simulink model "schSimuSegway_2020b"  (R2020b)
settings: Solver=VariableStepAuto  StartTime=0.0  StopTime=tfinal  RelTol=1e-3
InitFcn:
  | disp('init inports and outports numbers');
  | in_cb=1;
  | in_cm=2;
  | in_um=3;
  | out_thb=1;
  | out_thm=2;
  | out_vb=3;
  | out_vm=4;
  | out_um=5;
  | if exist('G')~=1
  | %--------------------------------------------------
  | % valeurs des parametres par defaut
  | %--------------------------------------------------
  | disp('init default parameters');
  | time_values_cb=[0,0];
  | time_values_cm=[0,0];
  | time_values_um=[0,0];
  | tfinal=10;
  | thm_init=0*pi/180;vthm_init=0*pi/180;
  | thb_init=0*pi/180;vthb_init=0*pi/180;
  | %------------------------------------------------------------------
  | % parametres des moteurs FIT0450U d'entrainement du segway en deplacement rectiligne
  | % dans ce cas les 2 moteurs sont attaques par la meme tension d'induit Um
  | %-----------------------------------------------------------------
  | 
  | Im=2*0.0061; % inertie de 2 moteurs en sortie de reducteur, ne devrait pas etre negligable !...
  | Kem= 0.277; % rapport fcem / vitesse en sortie de reducteur :V/(rd/s)=Nm/A;
  | 
  | Kim=2 *0.277;% 2. rapport couple  en sortie de reducteur/ courant :Nm/A = V/(rd/s);
  | Rm=2.8;% resistance d'induit en ohm
  | fm=2* 0.0108;% frottement visqueux en sortie de reducteur
  | u_max=5; % tension max des moteurs
  | u_dead=0.5; % bande morte due au frottement sec en volt
  | %------------------------------------------------------------------
  | % parametres mecanique du segway
  | %-----------------------------------------------------------------
  | G=9.81; % acceleration gravite terrestre en m/s2
  | % barre
  | Mb= 0.277; %Masse segway sans batterie 277g
  | Lb =  0.056000; % distance essieu centre de masse en m
  | Ib=1e-4 ; % inertie de la barre autour de son centre de masse en Kg.m^2
  | % batterie
  | Mbat=2*0.096; %masse en Kg des 2  batteries VoltCraft 5000 de 96g chacune
  | LxBat=0.022;LyBat=2*0.036;LzBat=0.075;
  | Ibat=1/12*Mbat*(LyBat^2+LzBat^2); % inertie batt/ centre de masse batt en kg.m2
  | Lbat=0.085;%0.085; % distance essieu centre de masse Batteries
  | %roues
  | Rr=0.07; % rayon des roues en m
  | Mr=2 * 0; % masse de 2 roues, negligable
  | Ir=1/2*Rr^2*Mr; % inertie des 2 roues, =1 cylindre plein de masse Mr, de rayon Rr autour de son axe de rotation
  | I1=Ir+(Mb+Mr+Mbat)*Rr^2; %avec Batterie
  | Ieb=Ib+Ibat+Mb*Lb^2+Mbat*Lbat^2;% avec Batterie
  | 
  | 
  | end
values from neighbouring files (symbols this model uses):
  Kem = 0.277    [programme_segway_etudiant.m]
settings Model: Creator=sygorra  LastModifiedBy=sygorra
settings DataIOCC: ReturnWorkspaceOutputs=off
settings DebuggingCC: ArithmeticOperatorsInVariantConditions=warning
settings SFSimCC: CustomCodeUndefinedFunction=UseInterfaceOnly

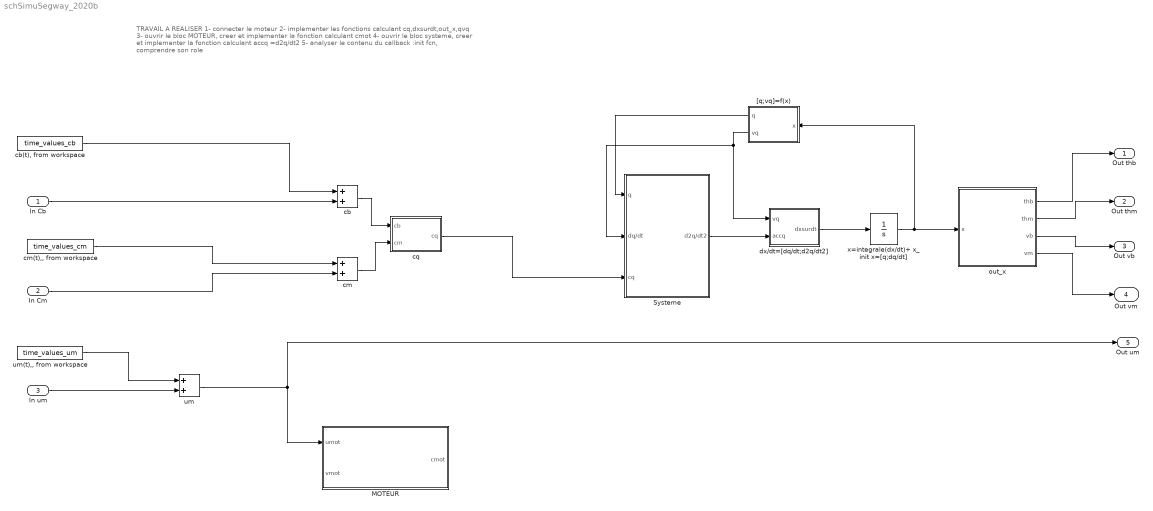
== system schSimuSegway_2020b ==
  note: TRAVAIL A REALISER
      | 1- connecter le moteur
      | 2- implementer les fonctions calculant cq,dxsurdt,out_x,qvq
      | 3- ouvrir le bloc MOTEUR, creer et implementer la fonction calculant cmot
      | 4- ouvrir le bloc systeme, creer et implementer la fonction calculant accq =d2q/dt2
      | 5- analyser le contenu du callback :init fcn, comprendre son role
  In Cb : Inport
  In Cm : Inport  Port=2
  In um : Inport  Port=3
  MOTEUR : Subsystem
  Systeme : Subsystem
  "[q;vq]=f(x)" : MATLAB Function  TreatAsAtomicUnit=on
  cb : Sum
  "cb(t), from workspace" : FromWorkspace  VariableName=time_values_cb
  cm : Sum
  "cm(t),, from workspace" : FromWorkspace  VariableName=time_values_cm
  cq : MATLAB Function  TreatAsAtomicUnit=on
  dx/dt=[dq/dt;d2q/dt2] : MATLAB Function  TreatAsAtomicUnit=on
  out_x : MATLAB Function  TreatAsAtomicUnit=on
  "um " : Sum
  "um(t),, from workspace" : FromWorkspace  VariableName=time_values_um
  x=integrale(dx/dt)+ x_init x=[q;dq/dt] : Integrator  InitialCondition=[thb_init;thm_init;vthb_init;vthm_init]
  Out thb : Outport  VectorParamsAs1DForOutWhenUnconnected=off
  Out thm : Outport  Port=2  VectorParamsAs1DForOutWhenUnconnected=off
  Out vb : Outport  Port=3  VectorParamsAs1DForOutWhenUnconnected=off
  Out vm : Outport  Port=4  VectorParamsAs1DForOutWhenUnconnected=off
  Out um : Outport  Port=5  VectorParamsAs1DForOutWhenUnconnected=off
  wires:
  "cb(t), from workspace"/1 -> cb/1
  In Cb/1 -> cb/2
  In um/1 -> "um "/2
  "um(t),, from workspace"/1 -> "um "/1
  In Cm/1 -> cm/2
  "cm(t),, from workspace"/1 -> cm/1
  cb/1 -> cq/1(cb)
  cm/1 -> cq/2(cm)
  cq/1(cq) -> Systeme/3(cq)
  x=integrale(dx/dt)+ x_init x=[q;dq/dt]/1 -> "[q;vq]=f(x)"/1(x), out_x/1(x)
  "[q;vq]=f(x)"/1(q) -> Systeme/1(q)
  "[q;vq]=f(x)"/2(vq) -> dx/dt=[dq/dt;d2q/dt2]/1(vq), Systeme/2(dq/dt)
  dx/dt=[dq/dt;d2q/dt2]/1(dxsurdt) -> x=integrale(dx/dt)+ x_init x=[q;dq/dt]/1
  Systeme/1(d2q/dt2) -> dx/dt=[dq/dt;d2q/dt2]/2(accq)
  out_x/1(thb) -> Out thb/1
  out_x/2(thm) -> Out thm/1
  out_x/3(vb) -> Out vb/1
  out_x/4(vm) -> Out vm/1
  "um "/1 -> Out um/1, MOTEUR/1(umot)

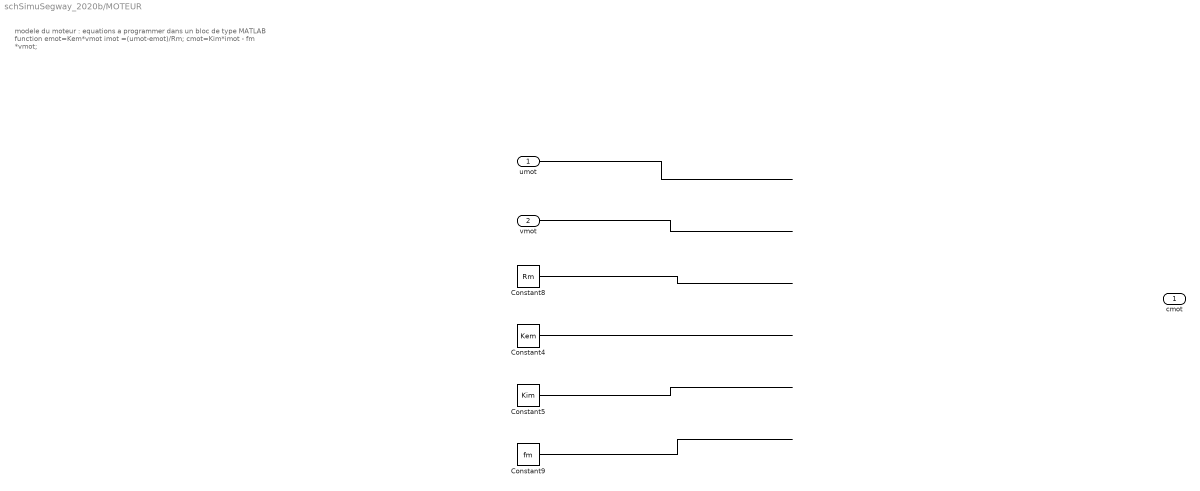
== system schSimuSegway_2020b/MOTEUR ==
  note: modele du moteur : equations a programmer dans un bloc de type MATLAB function
      | emot=Kem*vmot
      | imot =(umot-emot)/Rm;
      | cmot=Kim*imot - fm *vmot;
  umot : Inport
  vmot : Inport  Port=2
  Constant4 : Constant  Value=Kem
  Constant5 : Constant  Value=Kim
  Constant8 : Constant  Value=Rm
  Constant9 : Constant  Value=fm
  cmot : Outport
  wires:
  umot/1 -> ?
  Constant5/1 -> ?
  ? -> cmot/1
  Constant8/1 -> ?
  vmot/1 -> ?
  Constant4/1 -> ?
  Constant9/1 -> ?

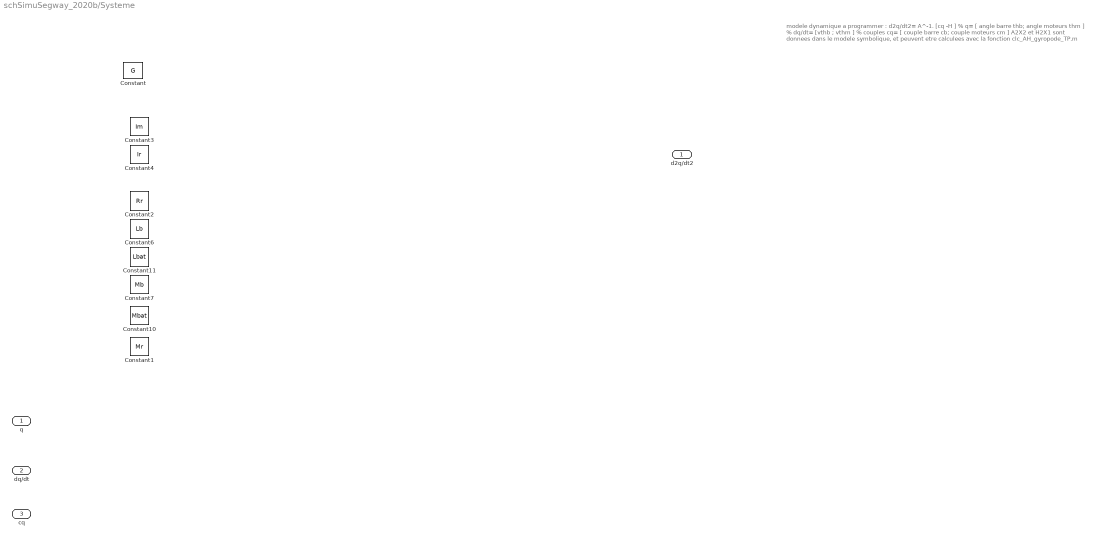
== system schSimuSegway_2020b/Systeme ==
  note: modele dynamique a programmer : d2q/dt2= A^-1. [cq -H ]
      |
      | % q= [ angle barre thb; angle moteurs thm ]
      | % dq/dt= [vthb ; vthm ]
      | % couples cq= [ couple barre cb; couple moteurs cm ]
      | A2X2 et H2X1 sont donnees dans le modele symbolique,
      | et peuvent etre calculees avec la fonction clc_AH_gyropode_TP.m
  q : Inport
  dq/dt : Inport  Port=2
  cq : Inport  Port=3
  Constant : Constant  Value=G
  Constant1 : Constant  Value=Mr
  Constant10 : Constant  Value=Mbat
  Constant11 : Constant  Value=Lbat
  Constant2 : Constant  Value=Rr
  Constant3 : Constant  Value=Im
  Constant4 : Constant  Value=Ir
  Constant6 : Constant  Value=Lb
  Constant7 : Constant  Value=Mb
  d2q/dt2 : Outport  VectorParamsAs1DForOutWhenUnconnected=off
  wires:
  ? -> d2q/dt2/1

== matlab function schSimuSegway_2020b/cq ==
  data: cb input; cq output; cm input
function cq =cq_(cb,cm)

cq=0;

== matlab function schSimuSegway_2020b/[q;vq]=f(x) ==
  data: x input; q output; vq output
function [q,vq] =qvq_(x)

q=0;
vq=0;

== matlab function schSimuSegway_2020b/dx//dt=[dq//dt;d2q//dt2] ==
  data: vq input; dxsurdt output; accq input
function dxsurdt  =vx_(vq,accq)

dxsurdt=0;

== matlab function schSimuSegway_2020b/out_x ==
  data: x input; thb output; thm output; vb output; vm output
function [thb,thm,vb,vm] =outputs_(x)

thb=0;
thm=0;
vthb=0;
vthm=0;
